simulink model "PubIfCommonEHRV2_MDL"  (R2020b)
settings: Solver=FixedStepAuto  StartTime=0.0  StopTime=Inf  RelTol=1e-3
PostLoadFcn:
  | if any(exist('dsrtsu_mdlpostloadfcn', 'file') ~= 0), dsrtsu_mdlpostloadfcn('Execute', bdroot); end
InitFcn:
  | , if any(exist('dsmpb_private', 'file') ~= 0), dsmpb_private('dsmpb_mdlclblib', 'Init', bdroot); end,
undefined symbols (not defined in the file): CAMERA_STATE_INITIAL, CAMERA_STATE_NORMAL, CURVATURE_UNKNOWN, DISTANCE_UNKONWN, DRIVING_ON_HIGHWAY_YES, EHR_CYCLE, FORWARD_LOOKING_DISTANCE_LIMIT, IFC_HUT_INTERFACE_NO_RESPONSE, IFC_HUT_INTERFACE_RESPONSE, MAP_DATA_VALID_VALID, MSG_TYPE_PROFILE_LONG, MSG_TYPE_PROFILE_SHORT, MSG_TYPE_SEGMENT, MSG_TYPE_STUB, OFFSET_INVALID, OFFSET_MAX, P_EHRV2_dCurvatureFar, P_EHRV2_dCurvatureMatrix, P_EHRV2_dSlopeFar, P_EHRV2_dSlopeMatrix, P_EHRV2_dVehForwardLooking, P_EHRV2_dVehRearLooking, P_EHRV2_tIFCHUTNoResponseOfForecastTreeReset, P_EHRV2_tIFCHUTNoResponseOfTimeout, P_EHRV2_tIFCHUTResponseTimeout, PROFILE_SHORT_NO_OTHER_VALUE, PROFILE_SHORT_TYPE_CURVATURE, PROFILE_SHORT_TYPE_SLOPE, REAR_LOOKING_DISTANCE_LIMIT, SLOPE_UNKNOWN, STUB_CMPLX_INSCT, STUB_FORM_OF_WAY_HIGH_RING_ROAD, STUB_FORM_OF_WAY_NORMAL_RING_ROAD
libraries: simulink x5
(part 3 of 4)

== matlab function PubIfCommonEHRV2_MDL/EHR/EHR_Main/DR_Calc_ProfileLongReconstruct ==
  data: PositionStruct input; ProfileLongVector input; RampInDistance output uint16; ProfileLongVectorSize input; MapDataValid input; DISTANCE_UNKONWN parameter; SPEED_LIMIT_UNKNOWN parameter; PROFILE_LONG_TYPE_TRAFFIC_SIGN parameter; PROFILE_LONG_VALUE_LANE_MERGE_RIGHT parameter; ElectronicEyeDistance output uint16; ElectronicEyeSpeedLimit output uint8; PROFILE_LONG_VALUE_ELECTRONIC_EYE parameter; SEGMENT_SPEED_LIMIT_5KMH parameter; SEGMENT_SPEED_LIMIT_7KMH parameter; SEGMENT_SPEED_LIMIT_UNLIMITED parameter; SPEED_LIMIT_UNLIMITED parameter; MAP_DATA_VALID_VALID parameter; TrafficSignDistance output uint16; TrafficSignValue output uint8; TRAFFIC_SIGN_UNKNOWN parameter; WeatherTypeValue output; WEATHER_TYPE_UNKNOWN parameter; PROFILE_LONG_TYPE_WEATHER_SIGN parameter; Temperature output; TEMPERATURE_UNKNOWN parameter; TrafficJamDistance output; TrafficJamDistanceHold output; PROFILE_LONG_TYPE_TRAFFIC_EVENT parameter; PROFILE_LONG_VALUE_TRAFFIC_JAM parameter; PROFILE_LONG_VALUE_REPAIR_ROAD_POINT parameter; RepairRoadPointDistance output; CtrlPointDistance output; StubRamp_dirc2 output; Stub_Type2 output; Ramp_Type2 output
 function [RampInDistance, ElectronicEyeDistance, ElectronicEyeSpeedLimit, TrafficSignDistance, ...
    TrafficSignValue, WeatherTypeValue, Temperature, TrafficJamDistance, TrafficJamDistanceHold,...
    RepairRoadPointDistance, CtrlPointDistance,StubRamp_dirc2,Stub_Type2,Ramp_Type2] = fcn(PositionStruct,...
    ProfileLongVector, ProfileLongVectorSize, MapDataValid, ...
    DISTANCE_UNKONWN, SPEED_LIMIT_UNKNOWN, PROFILE_LONG_TYPE_TRAFFIC_SIGN, PROFILE_LONG_VALUE_LANE_MERGE_RIGHT, PROFILE_LONG_VALUE_ELECTRONIC_EYE, SEGMENT_SPEED_LIMIT_5KMH, SEGMENT_SPEED_LIMIT_7KMH, SEGMENT_SPEED_LIMIT_UNLIMITED, SPEED_LIMIT_UNLIMITED, MAP_DATA_VALID_VALID, TRAFFIC_SIGN_UNKNOWN, WEATHER_TYPE_UNKNOWN, PROFILE_LONG_TYPE_WEATHER_SIGN, TEMPERATURE_UNKNOWN, PROFILE_LONG_TYPE_TRAFFIC_EVENT, PROFILE_LONG_VALUE_TRAFFIC_JAM, PROFILE_LONG_VALUE_REPAIR_ROAD_POINT)

%%%%Traffic Sign%%%%
t_flag_find_ramp_in = false;
t_flag_find_electronic_eye = false;
t_flag_find_traffic_sign = false;
t_flag_find_more_traffic_sign = false;

%%% Modify
t_flag_find_weather_sign = false;
t_flag_find_traffic_jam = false;
t_flag_find_repair_road_point = false;
t_flag_find_ctrl_point = false;

%%%
RampInDistance = DISTANCE_UNKONWN;
ElectronicEyeDistance = DISTANCE_UNKONWN;
ElectronicEyeSpeedLimit = SPEED_LIMIT_UNKNOWN;
TrafficSignDistance = DISTANCE_UNKONWN;
TrafficSignValue = TRAFFIC_SIGN_UNKNOWN;
TrafficSignRelativeOffset = int16(0);

WeatherTypeValue = WEATHER_TYPE_UNKNOWN;
Temperature = TEMPERATURE_UNKNOWN;
TrafficJamDistance = DISTANCE_UNKONWN;
TrafficJamDistanceHold = DISTANCE_UNKONWN;
RepairRoadPointDistance = DISTANCE_UNKONWN;
CtrlPointDistance = DISTANCE_UNKONWN;

StubRamp_dirc2 = uint8(0);
Stub_Type2 = uint8(0);
Ramp_Type2 = uint8(0);

%%%%overflow prevention%%%%
if (ProfileLongVectorSize == 0) || (MapDataValid ~= MAP_DATA_VALID_VALID)
    %Do nothing
else
    tWeatherK1 = uint16(1); %%%Modify 
    for t = 1:ProfileLongVectorSize
        %%%%Position Road%%%%
        if ProfileLongVector(t).ProfLongPathIdx == PositionStruct.PosnPathIdx
            %%%%Traffic Sign%%%%
            if ProfileLongVector(t).ProfLongProfType == PROFILE_LONG_TYPE_TRAFFIC_SIGN
                %%%%Signal TrafficSignDistance and TrafficSignValue%%%%
                if (false == t_flag_find_traffic_sign)    %If find new Traffic Sign, stop
                    if ProfileLongVector(t).ProfLongRelativeOffset < 0
                        TrafficSignDistance = DISTANCE_UNKONWN;
                        TrafficSignValue = TRAFFIC_SIGN_UNKNOWN;
                    else
                        if ProfileLongVector(t).ProfLongRelativeOffset > DISTANCE_UNKONWN
                            TrafficSignDistance = DISTANCE_UNKONWN;
                        else
                            TrafficSignDistance = uint16(ProfileLongVector(t).ProfLongRelativeOffset);
                        end

                        TrafficSignValue = EHR_Calc_TrafficSignValue(bitshift(ProfileLongVector(t).ProfLongValue,-24));
                        t_flag_find_traffic_sign = true;
                        TrafficSignRelativeOffset = ProfileLongVector(t).ProfLongRelativeOffset;
                    end
                else   %Some Traffic Sign at the same distance
                    if ProfileLongVector(t).ProfLongRelativeOffset == TrafficSignRelativeOffset
                        TrafficSignValue = min(TrafficSignValue,EHR_Calc_TrafficSignValue(bitshift(ProfileLongVector(t).ProfLongValue,-24)));
                    else
                        t_flag_find_more_traffic_sign = true;
                    end
                end
                %%%%Signal RampDistanceOut%%%%
                if (false == t_flag_find_ramp_in)...    %If find new Ramp In, stop
                && (bitshift(ProfileLongVector(t).ProfLongValue,-24) == PROFILE_LONG_VALUE_LANE_MERGE_RIGHT)   %From 32bit--39bit, High Byte
                    if(ProfileLongVector(t).ProfLongRelativeOffset < 0)
                        RampInDistance = DISTANCE_UNKONWN;
                    else
                        if(ProfileLongVector(t).ProfLongRelativeOffset > DISTANCE_UNKONWN)
                            RampInDistance = DISTANCE_UNKONWN;
                        else
                            RampInDistance = uint16(ProfileLongVector(t).ProfLongRelativeOffset);
                        end
    
                        t_flag_find_ramp_in = true;
                        StubRamp_dirc2 = uint8(1);
                        %走在主路上
                        Stub_Type2 = uint8(2);
                        Ramp_Type2 = uint8(5);
                    end
                    
                %%%%Signal ElectronicEyeDistance and l_ElectronicEyeSpeedLimit_ub%%%%
                elseif (false == t_flag_find_electronic_eye)...    %If find new Electronic Eye, stop
                    && (bitshift(ProfileLongVector(t).ProfLongValue,-24) == PROFILE_LONG_VALUE_ELECTRONIC_EYE)   %From 32bit--39bit, High Byte
                    if ProfileLongVector(t).ProfLongRelativeOffset < 0
                        ElectronicEyeDistance = DISTANCE_UNKONWN;
                        ElectronicEyeSpeedLimit = SPEED_LIMIT_UNKNOWN;
                    else
                        if ProfileLongVector(t).ProfLongRelativeOffset > DISTANCE_UNKONWN
                            ElectronicEyeDistance = DISTANCE_UNKONWN;
                        else
                            ElectronicEyeDistance = uint16(ProfileLongVector(t).ProfLongRelativeOffset);
                        end

                        ElectronicEyeSpeedLimit = EHR_Calc_SpeedLimit(bitand(bitshift(ProfileLongVector(t).ProfLongValue,-16),hex2dec('ff')));
                        t_flag_find_electronic_eye = true;
                    end
                else
                    %Do nothing
                end
                
            %%%    Modify    %%%
            %%%% Weather Type Value %%%%
            elseif ProfileLongVector(t).ProfLongProfType == PROFILE_LONG_TYPE_WEATHER_SIGN
                if (false == t_flag_find_weather_sign)...
                && (ProfileLongVector(tWeatherK1).ProfLongRelativeOffset  <= 0)...
                && (ProfileLongVector(t).ProfLongRelativeOffset > 0)...
                && (ProfileLongVector(tWeatherK1).ProfLongPathIdx == PositionStruct.PosnPathIdx)
            
                    WeatherTypeValue = uint8(bitshift(ProfileLongVector(t).ProfLongValue,-25));% High 7 bit.
                    Temperature = int8(bitshift(ProfileLongVector(t).ProfLongValue,-18) & 0x7f) - int8(63);
                    t_flag_find_weather_sign = true;
                    
                else
                    %Do nothing
                end
                
            %%%% Traffic Event Value %%%%
            elseif ProfileLongVector(t).ProfLongProfType == PROFILE_LONG_TYPE_TRAFFIC_EVENT
                %%%%Signal TrafficJamDistance%%%%
                if (false == t_flag_find_traffic_jam)...    %If find new Traffic Jam, stop
                && ((bitshift(ProfileLongVector(t).ProfLongValue,-19) & 0x7f) == PROFILE_LONG_VALUE_TRAFFIC_JAM)   %From 20bit--26bit
                    if(ProfileLongVector(t).ProfLongRelativeOffset < 0)
                        TrafficJamDistance = DISTANCE_UNKONWN;
                    else
                        if(ProfileLongVector(t).ProfLongRelativeOffset > DISTANCE_UNKONWN)
                            TrafficJamDistance = DISTANCE_UNKONWN;
                        else
                            TrafficJamDistance = uint16(ProfileLongVector(t).ProfLongRelativeOffset);
                        end
                        
                        t_flag_find_traffic_jam = true;
                    end
                end
                
                %%%%Signal RepairRoadPointDistance%%%%
                if (false == t_flag_find_repair_road_point)...    %If find new Repair Road Point, stop
                && ((bitshift(ProfileLongVector(t).ProfLongValue,-19) & 0x7f) == PROFILE_LONG_VALUE_REPAIR_ROAD_POINT)   %From 20bit--26bit
                    if(ProfileLongVector(t).ProfLongRelativeOffset < 0)
                        RepairRoadPointDistance = DISTANCE_UNKONWN;
                    else
                        if(ProfileLongVector(t).ProfLongRelativeOffset > DISTANCE_UNKONWN)
                            RepairRoadPointDistance = DISTANCE_UNKONWN;
                        else
                            RepairRoadPointDistance = uint16(ProfileLongVector(t).ProfLongRelativeOffset);
                        end
                        
                        t_flag_find_repair_road_point = true;
                    end
                end
                
                tWeatherK1 = t;
            end
            
            %%%%Ctrl Point%%%%
            if ProfileLongVector(t).ProfLongCtrlPoint == true
                %%%%Signal CtrlPointDistance%%%%
                if (false == t_flag_find_ctrl_point)    %If find new Ctrl Point, stop
                    if(ProfileLongVector(t).ProfLongRelativeOffset < 0)
                        CtrlPointDistance = DISTANCE_UNKONWN;
                    else
                        if(ProfileLongVector(t).ProfLongRelativeOffset > DISTANCE_UNKONWN)
                            CtrlPointDistance = DISTANCE_UNKONWN;
                        else
                            CtrlPointDistance = uint16(ProfileLongVector(t).ProfLongRelativeOffset);
                        end
                        
                        t_flag_find_ctrl_point = true;
                    end
                end
            end
            
            %%%  Modify   %%%%
        else
            %Do nothing
        end

        %%%%Break out of the cycle%%%%
        if (true == t_flag_find_ramp_in)...
        && (true == t_flag_find_electronic_eye)...
        && (true == t_flag_find_more_traffic_sign)...
        && (true == t_flag_find_weather_sign)...
        && (true == t_flag_find_traffic_jam)...
        && (true == t_flag_find_repair_road_point)...
        && (true == t_flag_find_ctrl_point)
            break;
        end
    end
end

== matlab function PubIfCommonEHRV2_MDL/EHR/EHR_Main/DR_Calc_ProfileShortReconstruct ==
  data: PositionStruct input; ProfileShortVector input; RoadCurvature output single; ProfileShortVectorSize input; MapDataValid input; PROFILE_SHORT_TYPE_CURVATURE parameter; PROFILE_SHORT_TYPE_SLOPE parameter; PROFILE_SHORT_NO_OTHER_VALUE parameter; DISTANCE_UNKONWN parameter; CURVATURE_UNKNOWN parameter; SLOPE_UNKNOWN parameter; RoadCurvatureFar output single; RoadCurvatureFarDistance output uint16; RoadSlope output single; RoadSlopeFar output single; MAP_DATA_VALID_VALID parameter; RoadCurvatureMatrix output single size=[10 2]; RoadCurvatureMatrixSize output uint8; RoadSlopeMatrix output single size=[10 2]; RoadSlopeMatrixSize output uint8; P_EHRV2_dCurvatureFar parameter; P_EHRV2_dSlopeFar parameter; P_EHRV2_dCurvatureMatrix parameter; P_EHRV2_dSlopeMatrix parameter
function [RoadCurvature, RoadCurvatureFar, RoadCurvatureFarDistance, RoadSlope, RoadSlopeFar,...
    RoadCurvatureMatrix, RoadCurvatureMatrixSize, RoadSlopeMatrix, RoadSlopeMatrixSize]...
    = fcn(PositionStruct,...
    ProfileShortVector, ProfileShortVectorSize, MapDataValid,...
    PROFILE_SHORT_TYPE_CURVATURE, PROFILE_SHORT_TYPE_SLOPE, PROFILE_SHORT_NO_OTHER_VALUE, DISTANCE_UNKONWN, CURVATURE_UNKNOWN, SLOPE_UNKNOWN, MAP_DATA_VALID_VALID, P_EHRV2_dCurvatureFar, P_EHRV2_dSlopeFar, P_EHRV2_dCurvatureMatrix, P_EHRV2_dSlopeMatrix)

%%%%Type Curvature%%%%
t_flag_find_road_curvature = false;

RoadCurvature = CURVATURE_UNKNOWN;
RoadCurvatureFar = CURVATURE_UNKNOWN;
RoadCurvatureFarDistance = DISTANCE_UNKONWN;

RoadCurvatureMatrix = single(zeros(10,2));
RoadCurvatureMatrixSize = uint8(0);

%%%%Type Slope%%%%
t_flag_find_road_slope = false;

RoadSlope = SLOPE_UNKNOWN;
RoadSlopeFar = SLOPE_UNKNOWN;

RoadSlopeMatrix = single(zeros(10,2));
RoadSlopeMatrixSize = uint8(0);

%%%%overflow prevention%%%%
if (ProfileShortVectorSize == 0) || (MapDataValid ~= MAP_DATA_VALID_VALID)
    %Do nothing
else
    tCurvatureK1 = uint16(1);
    tSlopeK1 = uint16(1);
    for t = 1:ProfileShortVectorSize
        if ProfileShortVector(t).ProfShortPathIdx == PositionStruct.PosnPathIdx
            %%%%Type Curvature%%%%
            if ProfileShortVector(t).ProfShortProfType == PROFILE_SHORT_TYPE_CURVATURE
                t_curvature_value0 = EHR_Calc_Curvature(ProfileShortVector(t).ProfShortValue0);%curvature value0 of t_iter
                t_curvature_value1 = EHR_Calc_Curvature(ProfileShortVector(t).ProfShortValue1);%curvature value1 of t_iter
                t_curvature_value0K1 = EHR_Calc_Curvature(ProfileShortVector(tCurvatureK1).ProfShortValue0);%curvature value0 of t_iterK1
                t_curvature_value1K1 = EHR_Calc_Curvature(ProfileShortVector(tCurvatureK1).ProfShortValue1);%curvature value1 of t_iterK1
                
                %%%%Signal RoadCurvature%%%%
                if (false == t_flag_find_road_curvature)...
                && (ProfileShortVector(t).ProfShortRelativeOffset <= 0)...
                && ((ProfileShortVector(t).ProfShortRelativeOffset + int16(ProfileShortVector(t).ProfShortDist1)) > 0)
                    RoadCurvature = t_curvature_value0;
                    t_flag_find_road_curvature = true;
                elseif (false == t_flag_find_road_curvature)...
                && ((ProfileShortVector(tCurvatureK1).ProfShortRelativeOffset + int16(ProfileShortVector(tCurvatureK1).ProfShortDist1)) <= 0)...
                && (ProfileShortVector(t).ProfShortRelativeOffset > 0)...
                && (ProfileShortVector(tCurvatureK1).ProfShortPathIdx == PositionStruct.PosnPathIdx)
                    RoadCurvature = t_curvature_value1K1;
                    if PROFILE_SHORT_NO_OTHER_VALUE == ProfileShortVector(tCurvatureK1).ProfShortDist1
                        RoadCurvature = t_curvature_value0K1;
                    end

                    t_flag_find_road_curvature = true;
                else
                    %Do nothing
                end
                
                %%%%Signal RoadCurvatureFar%%%%
                if (CURVATURE_UNKNOWN ~= t_curvature_value0)...
                && (ProfileShortVector(t).ProfShortRelativeOffset >= 0)...
                && (ProfileShortVector(t).ProfShortRelativeOffset <= P_EHRV2_dCurvatureFar)
                    if (CURVATURE_UNKNOWN == RoadCurvatureFar)...
                    || (abs(t_curvature_value0) > abs(RoadCurvatureFar))
                        RoadCurvatureFar = t_curvature_value0;
                        RoadCurvatureFarDistance = uint16(ProfileShortVector(t).ProfShortRelativeOffset);
                    else
                        %Do nothing
                    end
                end
                if (CURVATURE_UNKNOWN ~= t_curvature_value1)...
                && (PROFILE_SHORT_NO_OTHER_VALUE ~= ProfileShortVector(t).ProfShortDist1)...
                && ((ProfileShortVector(t).ProfShortRelativeOffset + int16(ProfileShortVector(t).ProfShortDist1)) >= 0)...
                && ((ProfileShortVector(t).ProfShortRelativeOffset + int16(ProfileShortVector(t).ProfShortDist1)) <= P_EHRV2_dCurvatureFar)
                    if (CURVATURE_UNKNOWN == RoadCurvatureFar)...
                    || (abs(t_curvature_value1) > abs(RoadCurvatureFar))
                        RoadCurvatureFar = t_curvature_value1;
                        RoadCurvatureFarDistance = uint16(ProfileShortVector(t).ProfShortRelativeOffset + int16(ProfileShortVector(t).ProfShortDist1));
                    else
                        %Do nothing
                    end
                end
                
                %%%%Signal RoadCurvatureMatrix%%%%
                if (ProfileShortVector(t).ProfShortRelativeOffset >= 0)...
                && (ProfileShortVector(t).ProfShortRelativeOffset <= P_EHRV2_dCurvatureMatrix)
                    RoadCurvatureMatrixSize = RoadCurvatureMatrixSize + 1;
                    if RoadCurvatureMatrixSize <= length(RoadCurvatureMatrix)
                        RoadCurvatureMatrix(RoadCurvatureMatrixSize,1) = t_curvature_value0;
                        RoadCurvatureMatrix(RoadCurvatureMatrixSize,2) = ProfileShortVector(t).ProfShortRelativeOffset;
                    else
                        RoadCurvatureMatrixSize = uint8(length(RoadCurvatureMatrix));
                    end
                end
                if (PROFILE_SHORT_NO_OTHER_VALUE ~= ProfileShortVector(t).ProfShortDist1)...
                && ((ProfileShortVector(t).ProfShortRelativeOffset + int16(ProfileShortVector(t).ProfShortDist1)) >= 0)...
                && ((ProfileShortVector(t).ProfShortRelativeOffset + int16(ProfileShortVector(t).ProfShortDist1)) <= P_EHRV2_dCurvatureMatrix)
                    RoadCurvatureMatrixSize = RoadCurvatureMatrixSize + 1;
                    if RoadCurvatureMatrixSize <= length(RoadCurvatureMatrix)
                        RoadCurvatureMatrix(RoadCurvatureMatrixSize,1) = t_curvature_value1;
                        RoadCurvatureMatrix(RoadCurvatureMatrixSize,2) = ProfileShortVector(t).ProfShortRelativeOffset + int16(ProfileShortVector(t).ProfShortDist1);
                    else
                        RoadCurvatureMatrixSize = uint8(length(RoadCurvatureMatrix));
                    end
                end
                tCurvatureK1 = t;
            end
            
            %%%%Type Slope%%%%
            if ProfileShortVector(t).ProfShortProfType == PROFILE_SHORT_TYPE_SLOPE 
                t_slope_value0 = EHR_Calc_Slope(ProfileShortVector(t).ProfShortValue0);%slope value0 of t_iter
                t_slope_value1 = EHR_Calc_Slope(ProfileShortVector(t).ProfShortValue1);%slope value1 of t_iter
                t_slope_value0K1 = EHR_Calc_Slope(ProfileShortVector(tSlopeK1).ProfShortValue0);%slope value0 of t_iterK1
                t_slope_value1K1 = EHR_Calc_Slope(ProfileShortVector(tSlopeK1).ProfShortValue1);%slope value1 of t_iterK1
                
                %%%%Signal RoadSlope%%%%
                if (false == t_flag_find_road_slope)...
                && (ProfileShortVector(t).ProfShortRelativeOffset <= 0)...
                && ((ProfileShortVector(t).ProfShortRelativeOffset + int16(ProfileShortVector(t).ProfShortDist1)) > 0)
                    RoadSlope = t_slope_value0;
                    t_flag_find_road_slope = true;
                elseif (false == t_flag_find_road_slope)...
                && ((ProfileShortVector(tSlopeK1).ProfShortRelativeOffset + int16(ProfileShortVector(tSlopeK1).ProfShortDist1)) <= 0)...
                && (ProfileShortVector(t).ProfShortRelativeOffset > 0)...
                && (ProfileShortVector(tSlopeK1).ProfShortPathIdx == PositionStruct.PosnPathIdx)
                    RoadSlope = t_slope_value1K1;
                    if PROFILE_SHORT_NO_OTHER_VALUE == ProfileShortVector(tSlopeK1).ProfShortDist1
                        RoadSlope = t_slope_value0K1;
                    end
                    t_flag_find_road_slope = true;
                else
                    %Do nothing
                end

                %%%%Signal RoadSlopeFar%%%%
                % (SLOPE_UNKNOWN ~= t_slope_value0)
                % && (ProfileShortVector(t).ProfShortRelativeOffset >= 0) Slope maybe not update in 60m
                if ProfileShortVector(t).ProfShortRelativeOffset <= P_EHRV2_dSlopeFar
                    RoadSlopeFar = t_slope_value0;
                end

                % && ((ProfileShortVector(t).ProfShortRelativeOffset + ProfileShortVector(t).ProfShortDist1) >= 0) Slope maybe not update in 60m 
                if (PROFILE_SHORT_NO_OTHER_VALUE ~= ProfileShortVector(t).ProfShortDist1)...
                && ((ProfileShortVector(t).ProfShortRelativeOffset + int16(ProfileShortVector(t).ProfShortDist1)) <= P_EHRV2_dSlopeFar)
                    RoadSlopeFar = t_slope_value1;
                end
                
                 %%%%Signal RoadSlopeMatrix%%%%
                 if (ProfileShortVector(t).ProfShortRelativeOffset >= 0)...
                 && (ProfileShortVector(t).ProfShortRelativeOffset <= P_EHRV2_dSlopeMatrix)
                    RoadSlopeMatrixSize = RoadSlopeMatrixSize + 1;
                    if RoadSlopeMatrixSize <= length(RoadSlopeMatrix)
                        RoadSlopeMatrix(RoadSlopeMatrixSize,1) = t_slope_value0;
                        RoadSlopeMatrix(RoadSlopeMatrixSize,2) = ProfileShortVector(t).ProfShortRelativeOffset;
                    else
                        RoadSlopeMatrixSize = uint8(length(RoadSlopeMatrix));
                    end
                 end
                 if (PROFILE_SHORT_NO_OTHER_VALUE ~= ProfileShortVector(t).ProfShortDist1)...
                 && ((ProfileShortVector(t).ProfShortRelativeOffset + int16(ProfileShortVector(t).ProfShortDist1)) >= 0)...
                 && ((ProfileShortVector(t).ProfShortRelativeOffset + int16(ProfileShortVector(t).ProfShortDist1)) <= P_EHRV2_dSlopeMatrix)
                    RoadSlopeMatrixSize = RoadSlopeMatrixSize + 1;
                    if RoadSlopeMatrixSize <= length(RoadSlopeMatrix)
                        RoadSlopeMatrix(RoadSlopeMatrixSize,1) = t_slope_value1;
                        RoadSlopeMatrix(RoadSlopeMatrixSize,2) = ProfileShortVector(t).ProfShortRelativeOffset + int16(ProfileShortVector(t).ProfShortDist1);
                    else
                        RoadSlopeMatrixSize = uint8(length(RoadSlopeMatrix));
                    end
                end
                 
                tSlopeK1 = t;
            end
        else
            %Do nothing
        end

        if (true == t_flag_find_road_curvature)...
        && (ProfileShortVector(t).ProfShortRelativeOffset > P_EHRV2_dCurvatureFar)...
        && (ProfileShortVector(t).ProfShortRelativeOffset > P_EHRV2_dCurvatureMatrix)...
        && (true == t_flag_find_road_slope)...
        && (ProfileShortVector(t).ProfShortRelativeOffset > P_EHRV2_dSlopeFar)...
        && (ProfileShortVector(t).ProfShortRelativeOffset > P_EHRV2_dSlopeMatrix)
            break;
        end
    end
end

== matlab function PubIfCommonEHRV2_MDL/EHR/EHR_Main/DR_Calc_RampDistance ==
  data: RampInDistance input; RampDistance output uint16; RampOutDistance input
function RampDistance  = fcn(RampInDistance, RampOutDistance)
if RampInDistance <= RampOutDistance
    RampDistance = RampInDistance;
else
    RampDistance = RampOutDistance;
end

== matlab function PubIfCommonEHRV2_MDL/EHR/EHR_Main/DR_Calc_SegmentReconstruct ==
  data: PositionStruct input; SegmentVector input; DrivingOnHighWay output uint8; SegmentVectorSize input; MapDataValid input; DRIVING_ON_HIGHWAY_UNKONWN parameter; SEGMENT_FUNC_ROAD_CLASS_EXPRESSWAY parameter; DRIVING_ON_HIGHWAY_YES parameter; DRIVING_ON_HIGHWAY_NO parameter; FormOfWay output uint8; EnterTunnelInfo output uint8; EnterBridgeInfo output uint8; NumOfLaneDrvDir output uint8; SpeedLimit output uint8; SpeedLimitType output; FORM_OF_WAY_UNKONWN parameter; SEGMENT_FORM_OF_WAY_MAIN_ROAD parameter; FORM_OF_WAY_YES parameter; FORM_OF_WAY_NO parameter; ENTER_TUNNEL_INFO_UNKONWN parameter; SEGMENT_IS_PART_OF_A_TUNNEL parameter; ENTER_TUNNEL_INFO_YES parameter; ENTER_TUNNEL_INFO_NO parameter; ENTER_BRIDGE_INFO_UNKONWN parameter; SEGMENT_IS_PART_OF_A_BRIDGE parameter; ENTER_BRIDGE_INFO_YES parameter; ENTER_BRIDGE_INFO_NO parameter; NUM_OF_LANE_DRIVER_DIRECTION_UNKNOWN parameter; SPEED_LIMIT_UNKNOWN parameter; SEGMENT_SPEED_LIMIT_5KMH parameter; SEGMENT_SPEED_LIMIT_7KMH parameter; SEGMENT_SPEED_LIMIT_UNLIMITED parameter; SPEED_LIMIT_UNLIMITED parameter; TunnelDistance output uint16; BridgeDistance output uint16; DISTANCE_UNKONWN parameter; MAP_DATA_VALID_VALID parameter; SEGMENT_FORM_OF_WAY_HIGH_RING_ROAD parameter; SEGMENT_FORM_OF_WAY_NORMAL_RING_ROAD parameter; FORM_OF_WAY_RING_ROAD parameter; FUNC_ROAD_CLASS_UNKNOWN parameter; FuncRoadClass output; BuildUpArea output; BUILD_UP_AREA_UNKNOWN parameter; SPEED_LIMIT_TYPE_UNKNOWN parameter; StubRamp_dirc3 output; Stub_Type3 output; Ramp_Type3 output; RampInDistance output; OnNavPath output
function [DrivingOnHighWay, FormOfWay, EnterTunnelInfo, EnterBridgeInfo, NumOfLaneDrvDir, SpeedLimit, SpeedLimitType, TunnelDistance, BridgeDistance, FuncRoadClass, BuildUpArea,StubRamp_dirc3,Stub_Type3,Ramp_Type3, RampInDistance,OnNavPath] = fcn(PositionStruct,...
    SegmentVector, SegmentVectorSize, MapDataValid,...
    DRIVING_ON_HIGHWAY_UNKONWN, SEGMENT_FUNC_ROAD_CLASS_EXPRESSWAY, DRIVING_ON_HIGHWAY_YES, DRIVING_ON_HIGHWAY_NO, FORM_OF_WAY_UNKONWN, SEGMENT_FORM_OF_WAY_MAIN_ROAD, FORM_OF_WAY_YES, FORM_OF_WAY_NO, ENTER_TUNNEL_INFO_UNKONWN, SEGMENT_IS_PART_OF_A_TUNNEL, ENTER_TUNNEL_INFO_YES, ENTER_TUNNEL_INFO_NO, ENTER_BRIDGE_INFO_UNKONWN, SEGMENT_IS_PART_OF_A_BRIDGE, ENTER_BRIDGE_INFO_YES, ENTER_BRIDGE_INFO_NO, NUM_OF_LANE_DRIVER_DIRECTION_UNKNOWN, SPEED_LIMIT_UNKNOWN, SEGMENT_SPEED_LIMIT_5KMH, SEGMENT_SPEED_LIMIT_7KMH, SEGMENT_SPEED_LIMIT_UNLIMITED, SPEED_LIMIT_UNLIMITED, DISTANCE_UNKONWN, MAP_DATA_VALID_VALID, SEGMENT_FORM_OF_WAY_HIGH_RING_ROAD, SEGMENT_FORM_OF_WAY_NORMAL_RING_ROAD, FORM_OF_WAY_RING_ROAD, FUNC_ROAD_CLASS_UNKNOWN, BUILD_UP_AREA_UNKNOWN, SPEED_LIMIT_TYPE_UNKNOWN)

%%%%Calculate data on current Position%%%%
t_flag_find_position = false;

DrivingOnHighWay = DRIVING_ON_HIGHWAY_UNKONWN;
FormOfWay = FORM_OF_WAY_UNKONWN;
EnterTunnelInfo = ENTER_TUNNEL_INFO_UNKONWN;
EnterBridgeInfo = ENTER_BRIDGE_INFO_UNKONWN;
NumOfLaneDrvDir = NUM_OF_LANE_DRIVER_DIRECTION_UNKNOWN;
SpeedLimit = SPEED_LIMIT_UNKNOWN;
SpeedLimitType = SPEED_LIMIT_TYPE_UNKNOWN;

%%%Modeify
FuncRoadClass = FUNC_ROAD_CLASS_UNKNOWN;
BuildUpArea = BUILD_UP_AREA_UNKNOWN;

%%%%Calculate data not on current position, for example, distance%%%%
t_flag_find_tunnel = false;
t_flag_find_bridge = false;
t_flag_find_ramp_in = false;

TunnelDistance = DISTANCE_UNKONWN;
BridgeDistance = DISTANCE_UNKONWN;

RampInDistance = DISTANCE_UNKONWN;
StubRamp_dirc3 = uint8(0);
Stub_Type3 = uint8(0);
Ramp_Type3 = uint8(0);
OnNavPath = uint8(0);
%%%%overflow prevention%%%%
if (SegmentVectorSize == 0) || (MapDataValid ~= MAP_DATA_VALID_VALID)
    OnNavPath = uint8(2);
else
    tK1 = uint16(1);
    for t = 1:SegmentVectorSize
        if SegmentVector(t).SegPathIdx == PositionStruct.PosnPathIdx
            %%%%%%
            if SegmentVector(t).SegPartOfCalcRoute == 1
                OnNavPath = uint8(1);
            else
                OnNavPath = uint8(0);
            end
            %%%%Calculate data on current Position%%%%
            if (false == t_flag_find_position)...
            && (SegmentVector(tK1).SegRelativeOffset <= 0)...
            && (SegmentVector(t).SegRelativeOffset > 0)...
            && (SegmentVector(tK1).SegPathIdx == PositionStruct.PosnPathIdx)
                %%%%%%%%%%%%%Signal DrivingOnHighWay%%%%%%%%%%%%%
                if SegmentVector(tK1).SegFuncRoadClass == SEGMENT_FUNC_ROAD_CLASS_EXPRESSWAY
                    DrivingOnHighWay = DRIVING_ON_HIGHWAY_YES;
                else
                    DrivingOnHighWay = DRIVING_ON_HIGHWAY_NO;
                end
                %%%%%%%%%%%%%Signal FormOfWay%%%%%%%%%%%%%
                if SegmentVector(tK1).SegFormOfWay == SEGMENT_FORM_OF_WAY_MAIN_ROAD
                    FormOfWay = FORM_OF_WAY_YES;
                elseif (SegmentVector(tK1).SegFormOfWay == SEGMENT_FORM_OF_WAY_HIGH_RING_ROAD)...
                    || (SegmentVector(tK1).SegFormOfWay == SEGMENT_FORM_OF_WAY_NORMAL_RING_ROAD)
                    FormOfWay = FORM_OF_WAY_RING_ROAD;
                else
                    FormOfWay = FORM_OF_WAY_NO;
                end
                %%%%%%%%%%%%%Signal EnterTunnelInfo%%%%%%%%%%%%%
                if SegmentVector(tK1).SegTunnel == SEGMENT_IS_PART_OF_A_TUNNEL
                    EnterTunnelInfo = ENTER_TUNNEL_INFO_YES;
                else
                    EnterTunnelInfo = ENTER_TUNNEL_INFO_NO;
                end
                %%%%%%%%%%%%%Signal EnterBridgeInfo%%%%%%%%%%%%%
                if SegmentVector(tK1).SegBridge == SEGMENT_IS_PART_OF_A_BRIDGE
                    EnterBridgeInfo = ENTER_BRIDGE_INFO_YES;
                else
                    EnterBridgeInfo = ENTER_BRIDGE_INFO_NO;
                end
                %%%%%%%%%%%%%Signal NumOfLaneDrvDir%%%%%%%%%%%%%
                NumOfLaneDrvDir = SegmentVector(tK1).SegNumOfLaneDrvDir;
                %%%%%%%%%%%%%Signal SpeedLimit%%%%%%%%%%%%%
                SpeedLimit = EHR_Calc_SpeedLimit(SegmentVector(tK1).SegEffSpdLmt);
                %%%%%%%%%%%%%Signal SpeedLimitType%%%%%%%%%%%%%
                SpeedLimitType = SegmentVector(tK1).SegEffSpdLmtType;
                %%%%%%%%%%%%%Signal FuncRoadClass%%%%%%%%%%%%%
                FuncRoadClass = SegmentVector(tK1).SegFuncRoadClass;
                %%%%%%%%%%%%%Signal BuildUpArea%%%%%%%%%%%%%
                BuildUpArea = SegmentVector(tK1).SegBuildUpArea;
                
                t_flag_find_position = true;
            else
                %Do nothing
            end
            
            %%%%Calculate data not on current position, for example, distance%%%%
            %%%%Calculate Tunnel Distance%%%%
            %%%%In tunnel%%%%
            if ENTER_TUNNEL_INFO_YES == EnterTunnelInfo
                TunnelDistance = uint16(0);
            %%%%Not in tunnel%%%%
            elseif (false == t_flag_find_tunnel)...    %If find new tunnel, stop
                     && (SegmentVector(t).SegTunnel == SEGMENT_IS_PART_OF_A_TUNNEL)
                %%%%Tunnel before position%%%%
                if SegmentVector(t).SegRelativeOffset < 0
                    TunnelDistance = DISTANCE_UNKONWN;
                %%%%Find new tunnel%%%%
                else
                    if SegmentVector(t).SegRelativeOffset > DISTANCE_UNKONWN
                        TunnelDistance = DISTANCE_UNKONWN;
                    else
                        TunnelDistance = uint16(SegmentVector(t).SegRelativeOffset);
                    end
                    t_flag_find_tunnel = true;
                end
            else
                %Do nothing
            end
            
            %%%%Calculate Bridge Distance%%%%
            if ENTER_BRIDGE_INFO_YES == EnterBridgeInfo
                BridgeDistance = uint16(0);
            %%%%Not in bridge%%%%
            elseif (false == t_flag_find_bridge)...    %If find new bridge, stop.
                     && (SegmentVector(t).SegBridge == SEGMENT_IS_PART_OF_A_BRIDGE)
                %%%%Bridge before position%%%%
                if SegmentVector(t).SegRelativeOffset < 0
                    BridgeDistance = DISTANCE_UNKONWN;
                %%%%Find new bridge%%%%
                else
                    if SegmentVector(t).SegRelativeOffset > DISTANCE_UNKONWN
                        BridgeDistance = DISTANCE_UNKONWN;
                    else
                        BridgeDistance = uint16(SegmentVector(t).SegRelativeOffset);
                    end
                    t_flag_find_bridge = true;
                end
            else
                %Do nothing
            end
            %%%%汇入%%%%
           if (false == t_flag_find_ramp_in)
                %%%%Tunnel before position%%%%
                if SegmentVector(t).SegRelativeOffset < 0
                    RampIntDistance = DISTANCE_UNKONWN;
                %%%%Find new tunnel%%%%
                end
                if SegmentVector(t).SegRelativeOffset > DISTANCE_UNKONWN
                        RampIntDistance = DISTANCE_UNKONWN;
                end
                [t_flag_find_ramp_in,RampInDistance,StubRamp_dirc3,Stub_Type3,Ramp_Type3] = RampIn_Judge(SegmentVector,SegmentVectorSize,PositionStruct,DISTANCE_UNKONWN);
            else
                %Do nothing
            end
            tK1 = t;
        else
            %Do nothing
        end

        %%%%Break out of the cycle%%%%
        if (true == t_flag_find_position) && (true == t_flag_find_tunnel) && (true == t_flag_find_bridge)
            break;
        end
    end
end

function  [t_flag_find_ramp_in_flag ,RampInDistance_flag ,StubRamp_dirc3_flag ,Stub_Type3_flag ,Ramp_Type3_flag ] = RampIn_Judge(SegmentVector,SegmentVectorSize,PositionStruct,DISTANCE_UNKONWN)
%%%%初始化%%%%
 SegmentVector_flag =  SegmentVector;
 ramp_flag = uint8(0);
 highway_flag = uint8(0);
 ramp_in = uint8(0);

t_flag_find_ramp_in_flag  = false;
RampInDistance_flag  = DISTANCE_UNKONWN;
StubRamp_dirc3_flag  = uint8(0);
Stub_Type3_flag  = uint8(0);
Ramp_Type3_flag  = uint8(0);
 %%%%查找是否存在匝道或是加速车道及高速路口%%%%
for m = 1:SegmentVectorSize
    if (SegmentVector_flag(m).SegFuncRoadClass ==4 || SegmentVector_flag(m).SegFuncRoadClass ==3) && SegmentVector_flag(m).SegFormOfWay==0
        ramp_flag = uint8(m);
    else
        ramp_flag = uint8(0);
    end
    if SegmentVector_flag(m).SegFuncRoadClass ==1 && SegmentVector_flag(m).SegFormOfWay == 2
        highway_flag = uint8(m);
    else
        highway_flag = uint8(0);
    end
end
%%%%如果存在匝道或是加速车道及高速路口%%%%
if ramp_flag > 0 && highway_flag > 0
    %%%%按照各segment距离排序%%%%
    for i = 1:SegmentVectorSize
        for j = i:SegmentVectorSize
            if SegmentVector_flag(i).SegOffset>SegmentVector_flag(j).SegOffset
                temp1 = SegmentVector_flag(j);
                SegmentVector_flag(j) = SegmentVector_flag(i);
                SegmentVector_flag(i) = temp1; 
            end
        end
    end
    for j = 1:SegmentVectorSize
        if ((SegmentVector_flag(j).SegFuncRoadClass ==4 || SegmentVector_flag(j).SegFuncRoadClass ==3) && SegmentVector_flag(j).SegFormOfWay==0) &&  (SegmentVector_flag(j+1).SegFuncRoadClass ==1 && SegmentVector_flag(j+1).SegFormOfWay == 2)
            ramp_in = uint8(j);
        else
            ramp_in = uint8(0);
        end
    end     
    if ramp_in>0
        t_flag_find_ramp_in_flag  = true;
        RampInDistance_flag  = SegmentVector_flag(ramp_in).SegOffset - PositionStruct.PosnOffset;
        StubRamp_dirc3_flag  = uint8(1);
        Stub_Type3_flag  = uint8(2);
        Ramp_Type3_flag  = uint8(4);
    end
end

== matlab function PubIfCommonEHRV2_MDL/EHR/EHR_Main/DR_Calc_StubReconstruct ==
  data: PositionStruct input; StubVector input; RampOutDistance output uint16; StubVectorSize input; MapDataValid input; DISTANCE_UNKONWN parameter; MAP_DATA_VALID_VALID parameter; RingRoadOutDistance output; STUB_FORM_OF_WAY_HIGH_RING_ROAD parameter; STUB_FORM_OF_WAY_NORMAL_RING_ROAD parameter; CmplxInsctDistance output; STUB_CMPLX_INSCT parameter; StubRamp_dirc1 output; Stub_Type1 output; Ramp_Type1 output; SegmentVector input
function [RampOutDistance, RingRoadOutDistance, CmplxInsctDistance,StubRamp_dirc1,Stub_Type1,Ramp_Type1]  = fcn(PositionStruct,...
    StubVector, StubVectorSize, MapDataValid, DISTANCE_UNKONWN, MAP_DATA_VALID_VALID, STUB_FORM_OF_WAY_HIGH_RING_ROAD, STUB_FORM_OF_WAY_NORMAL_RING_ROAD, STUB_CMPLX_INSCT,SegmentVector)

%%%%Calculate data not on current position, for example, distance%%%%
t_flag_find_ramp_out = false;
t_flag_find_ring_road_out = false;

%%%Modeify
t_flag_find_cmplx_insct = false;

RampOutDistance = DISTANCE_UNKONWN;%%630
RingRoadOutDistance = DISTANCE_UNKONWN;

%%%Modeify
CmplxInsctDistance = DISTANCE_UNKONWN;

StubRamp_dirc1 = uint8(0);
Stub_Type1 = uint8(0);
Ramp_Type1 = uint8(0);

%%%%overflow prevention%%%%
if (StubVectorSize == 0) || (MapDataValid ~= MAP_DATA_VALID_VALID)
    %Do nothing
else
    for t = 1:StubVectorSize
        if StubVector(t).StubPathIdx == PositionStruct.PosnPathIdx
            %%%%Calculate data not on current position, for example, distance%%%%
            %%%%Calculate Ramp Out Distance%%%%
            if (false == t_flag_find_ramp_out)    %If find new tunnel, stop
                %%%%Stub before position%%%%
                if StubVector(t).StubRelativeOffset < 0
                    RampOutDistance = DISTANCE_UNKONWN;
                %%%%Find new stub%%%%
                else
                    if StubVector(t).StubRelativeOffset > DISTANCE_UNKONWN
                        RampOutDistance = DISTANCE_UNKONWN;
                    else 
                        RampOutDistance = uint16(StubVector(t).StubRelativeOffset);
                    end
                        t_flag_find_ramp_out = true;
                        Stub_Type1 = uint8(1);
                        if RampOutDistance <500
                            StubRamp_dirc1 = Ramp_Dirc_Clc(StubVectorSize,StubVector);
                        end
                        
                        %高速到匝道
                        if (StubVector(t).StubFuncRoadClass == 1 || StubVector(t).StubFuncRoadClass==4) ...
                                && StubVector(t).StubFormOfWay == 0 && SegmentVector(t).SegFormOfWay == 2 
                            Ramp_Type1 = uint8(1);
                        end
                        %高速到高速
                        if StubVector(t).StubFuncRoadClass == 1 && StubVector(t).StubFormOfWay == 2 ...
                                && SegmentVector(t).SegFuncRoadClass == 1 && SegmentVector(t).SegFormOfWay == 2
                            Ramp_Type1 = uint8(2);
                        end
                         %匝道到匝道
                        if StubVector(t).StubFormOfWay == 0 && SegmentVector(t).SegFormOfWay == 0
                            Ramp_Type1 = uint8(3);
                        end
                end
               %%%%%%%
            else
                
            end
            %%%%Calculate Ring Road Out Distance%%%%
            if (false == t_flag_find_ring_road_out)    %If find new tunnel, stop
                if (StubVector(t).StubFormOfWay == STUB_FORM_OF_WAY_HIGH_RING_ROAD)...
                || (StubVector(t).StubFormOfWay == STUB_FORM_OF_WAY_NORMAL_RING_ROAD)
                    %%%%Ring road before position%%%%
                    if StubVector(t).StubRelativeOffset < 0
                        RingRoadOutDistance = DISTANCE_UNKONWN;
                    %%%%Find new ring road%%%%
                    else
                        if StubVector(t).StubRelativeOffset > DISTANCE_UNKONWN
                            RingRoadOutDistance = DISTANCE_UNKONWN;
                        else
                            RingRoadOutDistance = uint16(StubVector(t).StubRelativeOffset);
                        end
                        t_flag_find_ring_road_out = true;
                    end
                else
                end
            else
                %Do nothing
            end
            %%%%Calculate CmplxInsctDistance%%%%
            if (false == t_flag_find_cmplx_insct)...    %If find CmplxInsct, stop
            && (StubVector(t).StubCmplxInsct == STUB_CMPLX_INSCT)
                %%%%Stub before position%%%%
                if StubVector(t).StubRelativeOffset < 0
                    CmplxInsctDistance = DISTANCE_UNKONWN;
                %%%%Find new stub%%%%
                else
                    if StubVector(t).StubRelativeOffset > DISTANCE_UNKONWN
                        CmplxInsctDistance = DISTANCE_UNKONWN;
                    else
                        CmplxInsctDistance = uint16(StubVector(t).StubRelativeOffset);
                    end
                    t_flag_find_cmplx_insct = true;
                end
            else
                %Do nothing
            end
          
        else
            %Do nothing
        end

        %%%%Break out of the cycle%%%%
        if (true == t_flag_find_ramp_out)...
        && (true == t_flag_find_ring_road_out)...
        && (true == t_flag_find_cmplx_insct)...
            break;
        end
    end
    
    
    
end


function Ramp_dirc = Ramp_Dirc_Clc(StubVectorSize,StubVector)
Ramp_dirc = uint8(0);    
Idx_flag = uint16(0);
StubVector_flag = StubVector;
for i = 1:StubVectorSize
    for j = i:StubVectorSize
        if StubVector_flag(i).StubTurnAngl>StubVector_flag(j).StubTurnAngl
            temp1 = StubVector_flag(j).StubTurnAngl;
            StubVector_flag(j).StubTurnAngl = StubVector_flag(i).StubTurnAngl;
            StubVector_flag(i).StubTurnAngl = temp1; 

            temp2 = StubVector_flag(j).StubStubPathIdx;
            StubVector_flag(j).StubStubPathIdx = StubVector_flag(i).StubStubPathIdx;
            StubVector_flag(i).StubStubPathIdx =  temp2;    
        end
    end
end
for m = 1:StubVectorSize
    if StubVector_flag(m).StubStubPathIdx == uint16(6)
        Idx_flag = m;
    end
end
if  Idx_flag == 1 ||  StubVector_flag(Idx_flag).StubTurnAngl>180 
    Ramp_dirc = uint8(1);
end
if Idx_flag>1 && StubVector_flag(Idx_flag).StubTurnAngl<180
    Ramp_dirc = uint8(2);
end

== matlab function PubIfCommonEHRV2_MDL/EHR/EHR_Main/DS_Calc_ForecastTreeReset ==
  data: StubStruct input; StubStructK1 input; ForecastTreeResetFlag output boolean; OFFSET_INVALID parameter
function ForecastTreeResetFlag  = fcn(StubStruct, StubStructK1, ...
    OFFSET_INVALID)

if (StubStruct.StubCycCnt ~= StubStructK1.StubCycCnt)...   %Means this is a new message
&& (0 == StubStruct.StubPathIdx)...
&& (OFFSET_INVALID == StubStruct.StubOffset)
    ForecastTreeResetFlag = true;
else
    ForecastTreeResetFlag = false;
end

== matlab function PubIfCommonEHRV2_MDL/EHR/EHR_Main/DS_Calc_ProfileLongIsInDataWindow ==
  data: PositionStruct input; ProfileLongIsInDataWindow output boolean; ProfileLongStruct input; StubVector input; StubVectorSize input; P_EHRV2_dVehRearLooking parameter; P_EHRV2_dVehForwardLooking parameter
function ProfileLongIsInDataWindow = fcn(PositionStruct, ProfileLongStruct,...
    StubVector, StubVectorSize,...
    P_EHRV2_dVehRearLooking, P_EHRV2_dVehForwardLooking)

t_flag = false;  %Whether the valid stub data can be found

%%%%%%%%%Position Road%%%%%%%%%
if ProfileLongStruct.ProfLongPathIdx == PositionStruct.PosnPathIdx
    if (ProfileLongStruct.ProfLongRelativeOffset >= P_EHRV2_dVehRearLooking)...
        && (ProfileLongStruct.ProfLongRelativeOffset <= P_EHRV2_dVehForwardLooking)
        ProfileLongIsInDataWindow = true;
    else
        ProfileLongIsInDataWindow = false;
    end
%%%%%%%%%Other Road%%%%%%%%%
else
    %%%%iterator overflow prevention%%%%
    if 0 == StubVectorSize
        ProfileLongIsInDataWindow = false;
    else
       for t = 1:StubVectorSize
           if ProfileLongStruct.ProfLongPathIdx == StubVector(t).StubStubPathIdx
               t_flag = true;
               break;
           end
       end
       if true == t_flag   %This is stub
           ProfileLongIsInDataWindow = true;
       else
           ProfileLongIsInDataWindow = false;
       end
    end
end

== matlab function PubIfCommonEHRV2_MDL/EHR/EHR_Main/DS_Calc_ProfileLongIsUpdated ==
  data: ProfileLongStruct input; ProfileLongIsUpdated output boolean; ProfileLongVector input; ProfileLongVectorSize input
function ProfileLongIsUpdated = fcn(ProfileLongStruct, ProfileLongVector, ProfileLongVectorSize)

if 0 == ProfileLongStruct.ProfLongMsgType   %Means this struct is null
    ProfileLongIsUpdated = false;
else
    %%%%overflow prevention%%%%
    if 0 == ProfileLongVectorSize
        ProfileLongIsUpdated = true;
    elseif (ProfileLongStruct.ProfLongOffset == ProfileLongVector(ProfileLongVectorSize).ProfLongOffset)...
             && (ProfileLongStruct.ProfLongCycCnt == ProfileLongVector(ProfileLongVectorSize).ProfLongCycCnt)
        ProfileLongIsUpdated = false;
    else
        ProfileLongIsUpdated = true;
    end
end

== matlab function PubIfCommonEHRV2_MDL/EHR/EHR_Main/DS_Calc_ProfileLongVector ==
  data: PositionStruct input; ProfileLongVector output Bus: ProfileLongStruct size=50; PositionStructK1 input; ProfileLongStruct input; ProfileLongIsUpdated input; ProfileLongIsInDataWindow input; ForecastTreeResetFlag input; StubVector input; StubVectorSize input; ProfileLongVectorK1 input; ProfileLongVectorSizeK1 input; ProfileLongVectorSize output uint16; OFFSET_INVALID parameter; REAR_LOOKING_DISTANCE_LIMIT parameter; FORWARD_LOOKING_DISTANCE_LIMIT parameter; OFFSET_MAX parameter; P_EHRV2_dVehRearLooking parameter; P_EHRV2_dVehForwardLooking parameter
function [ProfileLongVector, ProfileLongVectorSize] = fcn(PositionStruct, PositionStructK1, ProfileLongStruct,...
    ProfileLongIsUpdated, ProfileLongIsInDataWindow, ForecastTreeResetFlag,...
    StubVector, StubVectorSize, ProfileLongVectorK1, ProfileLongVectorSizeK1,...
    OFFSET_INVALID, REAR_LOOKING_DISTANCE_LIMIT, FORWARD_LOOKING_DISTANCE_LIMIT, OFFSET_MAX, P_EHRV2_dVehRearLooking, P_EHRV2_dVehForwardLooking)

ProfileLongVector = ProfileLongVectorK1;
ProfileLongVectorSize = ProfileLongVectorSizeK1;

if true == ForecastTreeResetFlag
    for t = 1:ProfileLongVectorSize
        ProfileLongVector(t).ProfLongOffset = uint16(0);
        ProfileLongVector(t).ProfLongMsgType = uint8(0);
        ProfileLongVector(t).ProfLongPathIdx = uint8(0);
        ProfileLongVector(t).ProfLongCycCnt = uint8(0);
        ProfileLongVector(t).ProfLongUpdate = false;
        ProfileLongVector(t).ProfLongRetr = false;
        ProfileLongVector(t).ProfLongCtrlPoint = false;
        ProfileLongVector(t).ProfLongProfType = uint8(0);
        ProfileLongVector(t).ProfLongValue = uint32(0);
        ProfileLongVector(t).ProfLongRelativeOffset = int16(0);
    end
    ProfileLongVectorSize = uint16(0);
else
    %%%%%Update Actual Offset AND Delete%%%%%
    if (false == isequal(PositionStruct,PositionStructK1)) && (PositionStruct.PosnPathIdx > 3)   %Position is updated
        ProfileLongVectorSize = uint16(0);   %ProfileLongVectorSize need to be calculated again
        %%%%overflow prevention%%%%
        if 0 == ProfileLongVectorSizeK1
            %Do nothing
        else
            for t = 1:ProfileLongVectorSizeK1
                %%%%%Update Actual Offset%%%%%
                ProfileLongVector(t).ProfLongRelativeOffset = EHR_Calc_RelativeOffset(PositionStruct,ProfileLongVector(t).ProfLongPathIdx,ProfileLongVector(t).ProfLongOffset);
                %%%%%Delete%%%%%
                if DS_Calc_ProfileLongNeedDelete(PositionStruct,ProfileLongVector(t),P_EHRV2_dVehRearLooking,P_EHRV2_dVehForwardLooking,StubVector,StubVectorSize) == true
                    %Do nothing
                else
                    ProfileLongVectorSize = ProfileLongVectorSize + 1;
                    ProfileLongVector(ProfileLongVectorSize) = ProfileLongVector(t);
                end
            end
        end
    else
        %Do nothing
    end

    %%%%%Store%%%%%
    if (true == ProfileLongIsUpdated) && (true == ProfileLongIsInDataWindow) && (ProfileLongStruct.ProfLongPathIdx > 7)
        ProfileLongVectorSize = ProfileLongVectorSize + 1;
        if ProfileLongVectorSize <= length(ProfileLongVector)
            ProfileLongVector(ProfileLongVectorSize) = ProfileLongStruct;
        else
            ProfileLongVectorSize = uint16(length(ProfileLongVector));
        end
    else
        %Do nothing
    end

    if ProfileLongVectorSize < ProfileLongVectorSizeK1
        for t = (ProfileLongVectorSize + 1):ProfileLongVectorSizeK1
            ProfileLongVector(t).ProfLongOffset = uint16(0);
            ProfileLongVector(t).ProfLongMsgType = uint8(0);
            ProfileLongVector(t).ProfLongPathIdx = uint8(0);
            ProfileLongVector(t).ProfLongCycCnt = uint8(0);
            ProfileLongVector(t).ProfLongUpdate = false;
            ProfileLongVector(t).ProfLongRetr = false;
            ProfileLongVector(t).ProfLongCtrlPoint = false;
            ProfileLongVector(t).ProfLongProfType = uint8(0);
            ProfileLongVector(t).ProfLongValue = uint32(0);
            ProfileLongVector(t).ProfLongRelativeOffset = int16(0);
        end
    end
end
